simulink model "arm_static"  (R2025b)
settings: Solver=ode45  StartTime=0.0  StopTime=0.1  MaxStep=0.01  RelTol=1e-3
settings Model: Creator=Krishang  LastModifiedBy=Krishang

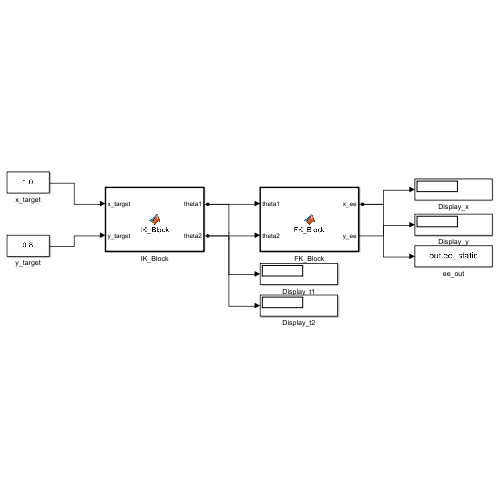
[thumbnail: Simulink's stored preview of the top-level diagram]
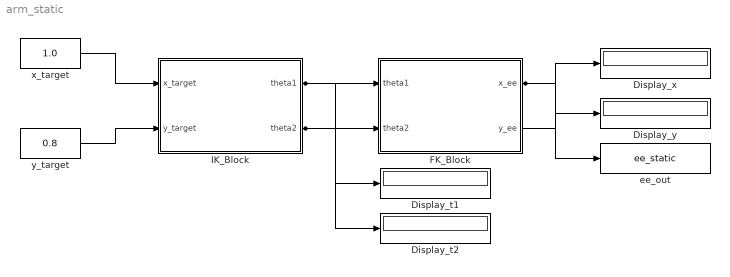
== system arm_static ==
  Display_t1 : Display
  Display_t2 : Display
  Display_x : Display
  Display_y : Display
  FK_Block : MATLAB Function  TreatAsAtomicUnit=on
  IK_Block : MATLAB Function  TreatAsAtomicUnit=on
  ee_out : ToWorkspace  VariableName=ee_static  SampleTime=-1
  x_target : Constant  Value=1.0
  y_target : Constant  Value=0.8
  wires:
  x_target/1 -> IK_Block/1(x_target)
  y_target/1 -> IK_Block/2(y_target)
  IK_Block/1(theta1) -> FK_Block/1(theta1), Display_t1/1
  IK_Block/2(theta2) -> FK_Block/2(theta2), Display_t2/1
  FK_Block/1(x_ee) -> Display_x/1, ee_out/1
  FK_Block/2(y_ee) -> Display_y/1

== matlab function arm_static/IK_Block ==
  data: x_target input; theta1 output; y_target input; theta2 output
function [theta1, theta2] = IK_Block(x_target, y_target)
L1 = 1.0; L2 = 0.8;
r     = sqrt(x_target^2 + y_target^2);
r_max = L1 + L2;
r_min = abs(L1 - L2);
r_s   = max(r_min + 1e-6, min(r_max - 1e-6, r));
if r > 1e-9
    xs = x_target * (r_s / r);
    ys = y_target * (r_s / r);
else
    xs = r_s; ys = 0;
end
c2     = max(-1, min(1, (xs^2 + ys^2 - L1^2 - L2^2) / (2*L1*L2)));
theta2 = atan2(sqrt(1 - c2^2), c2);
alpha  = atan2(ys, xs);
beta   = atan2(L2*sin(theta2), L1 + L2*cos(theta2));
theta1 = atan2(sin(alpha - beta), cos(alpha - beta));
end

== matlab function arm_static/FK_Block ==
  data: theta1 input; x_ee output; theta2 input; y_ee output
function [x_ee, y_ee] = FK_Block(theta1, theta2)
L1 = 1.0; L2 = 0.8;
x_ee = L1*cos(theta1) + L2*cos(theta1 + theta2);
y_ee = L1*sin(theta1) + L2*sin(theta1 + theta2);
end
